simulink model "sdrufreqcalib_rx"  (R2014a)
settings: Solver=FixedStepDiscrete  StartTime=0.0  StopTime=inf  RelTol=1e-3
libraries: sdrublksprivate x1, dspspect3 x1, commsdrhw_v2 x1
settings Model: SimulationMode=accelerator  Creator=The MathWorks Inc.
settings DataIOCC: SignalLoggingSaveFormat=ModelDataLogs
settings OptimizationCC: ExpressionDepthLimit=2147483647
settings DebuggingCC: UnderspecifiedInitializationDetection=Classic  ParameterPrecisionLossMsg=none  FcnCallInpInsideContextMsg=EnableAllAsWarning  StateNameClashWarn=warning
settings HardwareCC: TargetBitPerLong=64  TargetBitPerPointer=64  TargetLongLongMode=on  TargetIntDivRoundTo=Zero  TargetEndianess=LittleEndian  TargetWordSize=64  TargetHWDeviceType=Generic->MATLAB Host Computer  ProdEqTarget=off
settings RTWCC: CustomSourceCode=|
  | #include<stdio.h>
  | #include<stdlib.h>
settings GRTTargetCC: CombineOutputUpdateFcns=off  GRTInterface=on

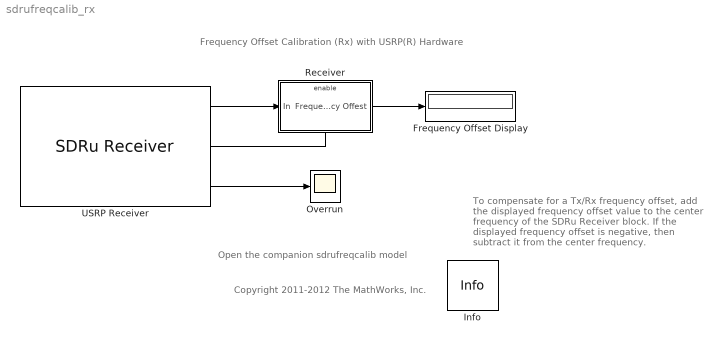
== system sdrufreqcalib_rx ==
  note: Frequency Offset Calibration (Rx)
      | with USRP(R) Hardware
  note: Open the companion sdrufreqcalib model
  note: Copyright 2011-2012 The MathWorks, Inc.
  note: To compensate for a Tx/Rx frequency offset,
      | add the displayed frequency offset value to the
      | center frequency of the SDRu Receiver block. If
      | the displayed frequency offset is negative, then
      | subtract it from the center frequency.
  Frequency Offset Display : Display
  Info : sdrublksprivate/Info  SystemSampleTime=-1
  Overrun : Scope
  Receiver : Subsystem
      mask Display: disp('Receiver')
  USRP Receiver : commsdrhw_v2/SDRu Receiver  rxtx=rx  USRP2_IP='192.168.10.2'  centerFrequency=900e6  centerFrequencySrc=Dialog  loOffset=0  loOffsetSrc=Dialog  gain=80  gainSrc=Dialog  decimInterp=5e2  decimInterpSrc=Dialog  USRP2_IP_NUM=[49 57 50 46 49 54 56 46 49 48 46 50]  frameLength=4096  outputDatatype=double  overrunUnderrunPort=on  sampleTime=1/2e5  HOST_DATA_PORT=0  HOST_CONTROL_PORT=0  USRP2_DATA_PORT=0  USRP2_CONTROL_PORT=0  bufferMode=Continuous streaming  EnableBurstMode=off  NumFramesInBurst=100
  wires:
  USRP Receiver/1 -> Receiver/1(In)
  USRP Receiver/2 -> Receiver/Enable
  USRP Receiver/3 -> Overrun/1
  Receiver/1(Frequency Offest) -> Frequency Offset Display/1

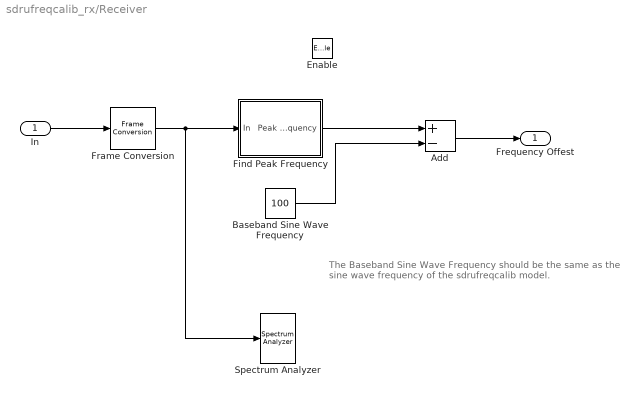
== system sdrufreqcalib_rx/Receiver ==
  note: The Baseband Sine Wave Frequency should be the same as
      | the sine wave frequency of the sdrufreqcalib model.
  In : Inport
  Enable : EnablePort
  Add : Sum  Inputs=+-
  Baseband Sine Wave Frequency : Constant  Value=100
  Find Peak Frequency : Subsystem
      mask Display: disp('Find Peak\nFrequency')
  Frame Conversion : FrameConversion
  Spectrum Analyzer : SpectrumAnalyzer
  Frequency Offest : Outport
  wires:
  In/1 -> Frame Conversion/1
  Frame Conversion/1 -> Find Peak Frequency/1(In), Spectrum Analyzer/1
  Find Peak Frequency/1(Peak Frequency) -> Add/1
  Baseband Sine Wave Frequency/1 -> Add/2
  Add/1 -> Frequency Offest/1

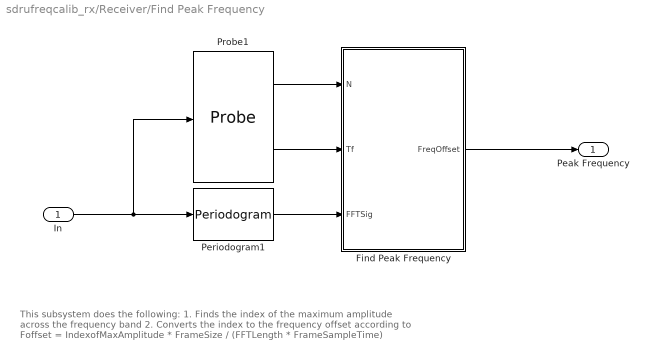
== system sdrufreqcalib_rx/Receiver/Find Peak Frequency ==
  note: This subsystem does the following:
      | 1.  Finds the index of the maximum amplitude across the frequency band
      | 2.  Converts the index to the frequency offset according to
      | Foffset = IndexofMaxAmplitude * FrameSize / (FFTLength * FrameSampleTime)
  In : Inport
  Find Peak Frequency : MATLAB Function  TreatAsAtomicUnit=on
  Periodogram1 : dspspect3/Periodogram  measurement=Power spectral density  wintype=Hamming  Rs=50  beta=5  winsamp=Symmetric  FFTImplementation=Auto  inheritFFT=off  fftsize=2048  navg=2  inheritTs=on  Ts=1
  Probe1 : Probe  ProbeComplexSignal=off
  Peak Frequency : Outport
  wires:
  Periodogram1/1 -> Find Peak Frequency/3(FFTSig)
  Probe1/1 -> Find Peak Frequency/1(N)
  Probe1/2 -> Find Peak Frequency/2(Tf)
  Find Peak Frequency/1(FreqOffset) -> Peak Frequency/1
  In/1 -> Periodogram1/1, Probe1/1

== matlab function sdrufreqcalib_rx/Receiver/Find Peak Frequency/Find Peak Frequency ==
  data: N input; FreqOffset output; Tf input; FFTSig input
function FreqOffset  = findpeakfreq(N, Tf, FFTSig)
% Find peak frequency
% N - frame size
% Tf - frame sample time
% FFTSig - result of FFT

%#codegen

FFTSize = length(FFTSig);
FFTSig = fftshift(FFTSig);
[~, maxIdx] = max(FFTSig); % Find index of max magnitude
OffsetIdx = maxIdx-1-FFTSize/2; % Convert to index symmetric with 0
Ts = Tf(1)/N; % Sample time
delta_f = 1/Ts/FFTSize; % Frequency resolution of FFT
FreqOffset = OffsetIdx*delta_f;% Map offset index back to frequency
